simulink model "s_deng_tvg_rev1_13_ramp"  (R2016b)
(part 2 of 19)

      mask prompts: max_pkt_len_bits "Max pkt length, 2^? 64-bit words"; header_ids "SPEAD direct address IDs (decimal)"; header_ind_ids "SPEAD indirect address IDs (decimal)"; spead_msw "SPEAD Flavour (MSw)"; spead_lsw "SPEAD Flavour (LSw)"; spead_version "SPEAD version"; bytes_per_word "Word size, in bytes"
      mask help:
      | This block generates SPEAD-compliant packets from a datastream.
      |
      | Packets are created with a fixed header followed by a number of 64-bit items.
      |
      | Requires a 64-bit data stream.
      |
      | The data_ready signal is one cycle BEFORE valid data! Does not have to be with a valid signal either.
      mask init:
      | if floor(log2(bytes_per_word)) ~= log2(bytes_per_word)
      |     error('Bytes per word should be a power of two.');
      | end
      | 
      | spead_pack_init(gcb)
  spead_pack3 : Subsystem  Tag=casper:spead_pack  AncestorBlock=casper_library_communications/spead_pack  mask(pkt_pack_mask){max_pkt_len_bits=10, header_ids=0x1600, 0x3101, 0x3102, header_ind_ids=0x3300, spead_msw=64, spead_lsw=48, spead_version=4, bytes_per_word=8}
      mask prompts: max_pkt_len_bits "Max pkt length, 2^? 64-bit words"; header_ids "SPEAD direct address IDs (decimal)"; header_ind_ids "SPEAD indirect address IDs (decimal)"; spead_msw "SPEAD Flavour (MSw)"; spead_lsw "SPEAD Flavour (LSw)"; spead_version "SPEAD version"; bytes_per_word "Word size, in bytes"
      mask help:
      | This block generates SPEAD-compliant packets from a datastream.
      |
      | Packets are created with a fixed header followed by a number of 64-bit items.
      |
      | Requires a 64-bit data stream.
      |
      | The data_ready signal is one cycle BEFORE valid data! Does not have to be with a valid signal either.
      mask init:
      | if floor(log2(bytes_per_word)) ~= log2(bytes_per_word)
      |     error('Bytes per word should be a power of two.');
      | end
      | 
      | spead_pack_init(gcb)
  spead_snap0 : Subsystem  Tag=casper:bitsnap  AncestorBlock=casper_library_scopes/bitfield_snapshot  mask(bitsnap){io_names=d64, io_widths=64, io_bps=0, io_types=0, show_format=on, snap_storage=bram, snap_dram_dimm=2, snap_dram_clock=250, snap_nsamples=15, snap_data_width=64, snap_offset=off, snap_circap=off, snap_value=off, snap_ext_arm=off, snap_ext_circ=off, snap_provide_outputs=on, snap_use_dsp48=on, snap_delay=2, extra_names=[c d], extra_widths=[30 2], extra_bps=[0 0], extra_types=[0 0]}
      mask prompts: io_names "Names [msb...lsb]"; io_widths "Bitwidths [msb...lsb]"; io_bps "Binary pts [msb...lsb]"; io_types "Data types [msb...lsb], ufix=0, fix=1, bool=2"; show_format "Print format string?"; snap_storage "Storage medium"; snap_dram_dimm "DRAM dimm"; snap_dram_clock "DRAM clock rate"; snap_nsamples "Number of Samples (2^?)"; snap_data_width "Data width"; snap_offset "Start delay support"; snap_circap "Circular capture support"; snap_value "Extra value capture support"; snap_ext_arm "External arm support"; snap_ext_circ "External circular capture support"; snap_provide_outputs "Provide outputs"; snap_use_dsp48 "Use DSP48s to implement counters"; snap_delay "Pre-snapshot delay"; extra_names "Names [msb...lsb]"; extra_widths "Widths [msb...lsb]"; extra_bps "Binary pts [msb...lsb]"; extra_types "Data types [msb...lsb], ufix=0, fix=1, bool=2"
      mask help:
      | A wrapped snapshot block. Allows specification of inputs to a snapblock word so the toolflow can automatically set up the scope.
      | See documentation for snapshot for explanation of parameters.
      mask init:
      | bitsnap_init(gcb);
      settings: AttributesFormatString=|
      | snap(1):uf64.0 = 64 bits\n64 wide, 32768 deep
      | debugID: 92947725
      mask TypeOptions snap_storage: bram | dram
      mask Callback snap_storage: bitsnap_callback();
      mask TypeOptions snap_dram_dimm: 1 | 2 | 3 | 4
      mask TypeOptions snap_dram_clock: 200 | 250 | 266 | 300 | 333
      mask TypeOptions snap_data_width: 8 | 16 | 32 | 64 | 128
      mask Callback snap_value: bitsnap_callback();
      mask Callback snap_ext_arm: bitsnap_callback();
      mask Callback snap_ext_circ: bitsnap_callback();
      mask Callback snap_provide_outputs: bitsnap_callback();
  speadsnap_control : Subsystem  Tag=xps:sw_reg  AncestorBlock=xps_library/software_register  mask(swreg){io_dir=From Processor, io_delay=0, sample_period=1, names=[speadsnap_arm], bitwidths=1, bin_pts=0, arith_types=2, sim_port=off, show_format=on}
      mask prompts: io_dir "I/O direction"; io_delay "I/O delay"; sample_period "Sample period"; names "Bitfield names [msb...lsb]"; bitwidths "Bitfield widths"; bin_pts "Bitfield binary pts"; arith_types "Bitfield types, ufix=0, fix=1, bool=2"; sim_port "Provide sim input/output?"; show_format "Print format string?"
      mask help: A 32-bit software-accessible register. Can be divided into bitfields of varying widths and types using the fields in the block mask.
      mask init:
      | swreg_init(gcb)
      settings: AttributesFormatString=1input:b = 1 bits
      mask TypeOptions io_dir: To Processor | From Processor
      mask Callback io_dir:
      | mask_enables = get_param(gcb, 'MaskEnables');
      | mask_names = get_param(gcb, 'MaskNames');
      | if strcmp(get_param(gcb, 'io_dir'), 'To Processor'),
      |     mask_enables{ismember(mask_names, 'sample_period')} = 'off';
      | else
      |     mask_enables{ismember(mask_names, 'sample_period')} = 'on';
      | end
      | set_param(gcb, 'MaskEnables', mask_enables);
  speadtime0_offset : Subsystem  Tag=xps:sw_reg  AncestorBlock=xps_library/software register  mask(swreg){io_dir=From Processor, io_delay=1, sample_period=1, names=speadtime_offset0, bitwidths=32, bin_pts=0, arith_types=0, sim_port=on, show_format=on}
      mask prompts: io_dir "I/O direction"; io_delay "I/O delay"; sample_period "Sample period"; names "Bitfield names [msb...lsb]"; bitwidths "Bitfield widths"; bin_pts "Bitfield binary pts"; arith_types "Bitfield types, ufix=0, fix=1, bool=2"; sim_port "Provide sim input/output?"; show_format "Print format string?"
      mask help: A 32-bit software-accessible register. Can be divided into bitfields of varying widths and types using the fields in the block mask.
      mask init:
      | try
      |     swreg_init(gcb)
      | catch ex
      |     disp(sprintf('%s: %s', gcb, ex.message))
      |     errordlg(ex.message)
      | end
      settings: AttributesFormatString=1input:uf32.0 = 32 bits
      mask TypeOptions io_dir: To Processor | From Processor
      mask Callback io_dir:
      | mask_enables = get_param(gcb, 'MaskEnables');
      | mask_names = get_param(gcb, 'MaskNames');
      | if strcmp(get_param(gcb, 'io_dir'), 'To Processor'),
      |     mask_enables{ismember(mask_names, 'sample_period')} = 'off';
      | else
      |     mask_enables{ismember(mask_names, 'sample_period')} = 'on';
      | end
      | set_param(gcb, 'MaskEnables', mask_enables);
  speadtime1_offset : Subsystem  Tag=xps:sw_reg  AncestorBlock=xps_library/software register  mask(swreg){io_dir=From Processor, io_delay=1, sample_period=1, names=speadtime_offset1, bitwidths=32, bin_pts=0, arith_types=0, sim_port=on, show_format=on}
      mask prompts: io_dir "I/O direction"; io_delay "I/O delay"; sample_period "Sample period"; names "Bitfield names [msb...lsb]"; bitwidths "Bitfield widths"; bin_pts "Bitfield binary pts"; arith_types "Bitfield types, ufix=0, fix=1, bool=2"; sim_port "Provide sim input/output?"; show_format "Print format string?"
      mask help: A 32-bit software-accessible register. Can be divided into bitfields of varying widths and types using the fields in the block mask.
      mask init:
      | try
      |     swreg_init(gcb)
      | catch ex
      |     disp(sprintf('%s: %s', gcb, ex.message))
      |     errordlg(ex.message)
      | end
      settings: AttributesFormatString=1input:uf32.0 = 32 bits
      mask TypeOptions io_dir: To Processor | From Processor
      mask Callback io_dir:
      | mask_enables = get_param(gcb, 'MaskEnables');
      | mask_names = get_param(gcb, 'MaskNames');
      | if strcmp(get_param(gcb, 'io_dir'), 'To Processor'),
      |     mask_enables{ismember(mask_names, 'sample_period')} = 'off';
      | else
      |     mask_enables{ismember(mask_names, 'sample_period')} = 'on';
      | end
      | set_param(gcb, 'MaskEnables', mask_enables);
  start_flag_lsw : Subsystem  Tag=xps:sw_reg  AncestorBlock=xps_library/software register  mask(swreg){io_dir=From Processor, io_delay=1, sample_period=1, names=reg, bitwidths=32, bin_pts=0, arith_types=0, sim_port=on, show_format=on}
      mask prompts: io_dir "I/O direction"; io_delay "I/O delay"; sample_period "Sample period"; names "Bitfield names [msb...lsb]"; bitwidths "Bitfield widths"; bin_pts "Bitfield binary pts"; arith_types "Bitfield types, ufix=0, fix=1, bool=2"; sim_port "Provide sim input/output?"; show_format "Print format string?"
      mask help: A 32-bit software-accessible register. Can be divided into bitfields of varying widths and types using the fields in the block mask.
      mask init:
      | try
      |     swreg_init(gcb)
      | catch ex
      |     disp(sprintf('%s: %s', gcb, ex.message))
      |     errordlg(ex.message)
      | end
      settings: AttributesFormatString=1input:uf32.0 = 32 bits
      mask TypeOptions io_dir: To Processor | From Processor
      mask Callback io_dir:
      | mask_enables = get_param(gcb, 'MaskEnables');
      | mask_names = get_param(gcb, 'MaskNames');
      | if strcmp(get_param(gcb, 'io_dir'), 'To Processor'),
      |     mask_enables{ismember(mask_names, 'sample_period')} = 'off';
      | else
      |     mask_enables{ismember(mask_names, 'sample_period')} = 'on';
      | end
      | set_param(gcb, 'MaskEnables', mask_enables);
  start_flag_msw : Subsystem  Tag=xps:sw_reg  AncestorBlock=xps_library/software register  mask(swreg){io_dir=From Processor, io_delay=1, sample_period=1, names=reg, bitwidths=32, bin_pts=0, arith_types=0, sim_port=on, show_format=on}
      mask prompts: io_dir "I/O direction"; io_delay "I/O delay"; sample_period "Sample period"; names "Bitfield names [msb...lsb]"; bitwidths "Bitfield widths"; bin_pts "Bitfield binary pts"; arith_types "Bitfield types, ufix=0, fix=1, bool=2"; sim_port "Provide sim input/output?"; show_format "Print format string?"
      mask help: A 32-bit software-accessible register. Can be divided into bitfields of varying widths and types using the fields in the block mask.
      mask init:
      | try
      |     swreg_init(gcb)
      | catch ex
      |     disp(sprintf('%s: %s', gcb, ex.message))
      |     errordlg(ex.message)
      | end
      settings: AttributesFormatString=1input:uf32.0 = 32 bits
      mask TypeOptions io_dir: To Processor | From Processor
      mask Callback io_dir:
      | mask_enables = get_param(gcb, 'MaskEnables');
      | mask_names = get_param(gcb, 'MaskNames');
      | if strcmp(get_param(gcb, 'io_dir'), 'To Processor'),
      |     mask_enables{ismember(mask_names, 'sample_period')} = 'off';
      | else
      |     mask_enables{ismember(mask_names, 'sample_period')} = 'on';
      | end
      | set_param(gcb, 'MaskEnables', mask_enables);
  start_time_lsw : Subsystem  Tag=xps:sw_reg  AncestorBlock=xps_library/software register  mask(swreg){io_dir=From Processor, io_delay=1, sample_period=1, names=reg, bitwidths=32, bin_pts=0, arith_types=0, sim_port=on, show_format=on}
      mask prompts: io_dir "I/O direction"; io_delay "I/O delay"; sample_period "Sample period"; names "Bitfield names [msb...lsb]"; bitwidths "Bitfield widths"; bin_pts "Bitfield binary pts"; arith_types "Bitfield types, ufix=0, fix=1, bool=2"; sim_port "Provide sim input/output?"; show_format "Print format string?"
      mask help: A 32-bit software-accessible register. Can be divided into bitfields of varying widths and types using the fields in the block mask.
      mask init:
      | try
      |     swreg_init(gcb)
      | catch ex
      |     disp(sprintf('%s: %s', gcb, ex.message))
      |     errordlg(ex.message)
      | end
      settings: AttributesFormatString=1input:uf32.0 = 32 bits
      mask TypeOptions io_dir: To Processor | From Processor
      mask Callback io_dir:
      | mask_enables = get_param(gcb, 'MaskEnables');
      | mask_names = get_param(gcb, 'MaskNames');
      | if strcmp(get_param(gcb, 'io_dir'), 'To Processor'),
      |     mask_enables{ismember(mask_names, 'sample_period')} = 'off';
      | else
      |     mask_enables{ismember(mask_names, 'sample_period')} = 'on';
      | end
      | set_param(gcb, 'MaskEnables', mask_enables);
  start_time_msw : Subsystem  Tag=xps:sw_reg  AncestorBlock=xps_library/software register  mask(swreg){io_dir=From Processor, io_delay=1, sample_period=1, names=reg, bitwidths=32, bin_pts=0, arith_types=0, sim_port=on, show_format=on}
      mask prompts: io_dir "I/O direction"; io_delay "I/O delay"; sample_period "Sample period"; names "Bitfield names [msb...lsb]"; bitwidths "Bitfield widths"; bin_pts "Bitfield binary pts"; arith_types "Bitfield types, ufix=0, fix=1, bool=2"; sim_port "Provide sim input/output?"; show_format "Print format string?"
      mask help: A 32-bit software-accessible register. Can be divided into bitfields of varying widths and types using the fields in the block mask.
      mask init:
      | try
      |     swreg_init(gcb)
      | catch ex
      |     disp(sprintf('%s: %s', gcb, ex.message))
      |     errordlg(ex.message)
      | end
      settings: AttributesFormatString=1input:uf32.0 = 32 bits
      mask TypeOptions io_dir: To Processor | From Processor
      mask Callback io_dir:
      | mask_enables = get_param(gcb, 'MaskEnables');
      | mask_names = get_param(gcb, 'MaskNames');
      | if strcmp(get_param(gcb, 'io_dir'), 'To Processor'),
      |     mask_enables{ismember(mask_names, 'sample_period')} = 'off';
      | else
      |     mask_enables{ismember(mask_names, 'sample_period')} = 'on';
      | end
      | set_param(gcb, 'MaskEnables', mask_enables);
  test_control : Subsystem  Tag=xps:sw_reg  AncestorBlock=xps_library/software_register  mask(swreg){io_dir=From Processor, io_delay=0, sample_period=1, names=[sel_ramp80 rst_ramp80 sel_munge], bitwidths=1, bin_pts=0, arith_types=2, sim_port=off, show_format=on}
      mask prompts: io_dir "I/O direction"; io_delay "I/O delay"; sample_period "Sample period"; names "Bitfield names [msb...lsb]"; bitwidths "Bitfield widths"; bin_pts "Bitfield binary pts"; arith_types "Bitfield types, ufix=0, fix=1, bool=2"; sim_port "Provide sim input/output?"; show_format "Print format string?"
      mask help: A 32-bit software-accessible register. Can be divided into bitfields of varying widths and types using the fields in the block mask.
      mask init:
      | swreg_init(gcb)
      settings: AttributesFormatString=3 inputs:b,b,b = 3 bits
      mask TypeOptions io_dir: To Processor | From Processor
      mask Callback io_dir:
      | mask_enables = get_param(gcb, 'MaskEnables');
      | mask_names = get_param(gcb, 'MaskNames');
      | if strcmp(get_param(gcb, 'io_dir'), 'To Processor'),
      |     mask_enables{ismember(mask_names, 'sample_period')} = 'off';
      | else
      |     mask_enables{ismember(mask_names, 'sample_period')} = 'on';
      | end
      | set_param(gcb, 'MaskEnables', mask_enables);
  tick_offset_lsw : Subsystem  Tag=xps:sw_reg  AncestorBlock=xps_library/software register  mask(swreg){io_dir=From Processor, io_delay=1, sample_period=1, names=reg, bitwidths=32, bin_pts=0, arith_types=0, sim_port=off, show_format=on}
      mask prompts: io_dir "I/O direction"; io_delay "I/O delay"; sample_period "Sample period"; names "Bitfield names [msb...lsb]"; bitwidths "Bitfield widths"; bin_pts "Bitfield binary pts"; arith_types "Bitfield types, ufix=0, fix=1, bool=2"; sim_port "Provide sim input/output?"; show_format "Print format string?"
      mask help: A 32-bit software-accessible register. Can be divided into bitfields of varying widths and types using the fields in the block mask.
      mask init:
      | try
      |     swreg_init(gcb)
      | catch ex
      |     disp(sprintf('%s: %s', gcb, ex.message))
      |     errordlg(ex.message)
      | end
      settings: AttributesFormatString=1input:uf32.0 = 32 bits
      mask TypeOptions io_dir: To Processor | From Processor
      mask Callback io_dir:
      | mask_enables = get_param(gcb, 'MaskEnables');
      | mask_names = get_param(gcb, 'MaskNames');
      | if strcmp(get_param(gcb, 'io_dir'), 'To Processor'),
      |     mask_enables{ismember(mask_names, 'sample_period')} = 'off';
      | else
      |     mask_enables{ismember(mask_names, 'sample_period')} = 'on';
      | end
      | set_param(gcb, 'MaskEnables', mask_enables);
  tick_offset_msw : Subsystem  Tag=xps:sw_reg  AncestorBlock=xps_library/software register  mask(swreg){io_dir=From Processor, io_delay=1, sample_period=1, names=reg, bitwidths=32, bin_pts=0, arith_types=0, sim_port=off, show_format=on}
      mask prompts: io_dir "I/O direction"; io_delay "I/O delay"; sample_period "Sample period"; names "Bitfield names [msb...lsb]"; bitwidths "Bitfield widths"; bin_pts "Bitfield binary pts"; arith_types "Bitfield types, ufix=0, fix=1, bool=2"; sim_port "Provide sim input/output?"; show_format "Print format string?"
      mask help: A 32-bit software-accessible register. Can be divided into bitfields of varying widths and types using the fields in the block mask.
      mask init:
      | try
      |     swreg_init(gcb)
      | catch ex
      |     disp(sprintf('%s: %s', gcb, ex.message))
      |     errordlg(ex.message)
      | end
      settings: AttributesFormatString=1input:uf32.0 = 32 bits
      mask TypeOptions io_dir: To Processor | From Processor
      mask Callback io_dir:
      | mask_enables = get_param(gcb, 'MaskEnables');
      | mask_names = get_param(gcb, 'MaskNames');
      | if strcmp(get_param(gcb, 'io_dir'), 'To Processor'),
      |     mask_enables{ismember(mask_names, 'sample_period')} = 'off';
      | else
      |     mask_enables{ismember(mask_names, 'sample_period')} = 'on';
      | end
      | set_param(gcb, 'MaskEnables', mask_enables);
  ticks_since_mrst : Subsystem
  tvg_spead_time_with_pkt_ctr : Subsystem  mask{packetlen_bits=9}
      mask prompts: packetlen_bits "Packet length, num 80-bit words (2^?):"
  wr_addr{0..3} (4 alike) : xbsIndex_r4/Counter  cnt_type=Free Running  cnt_to=Inf  operation=Up  start_count=0  cnt_by_val=1  arith_type=Unsigned  n_bits=10  bin_pt=0  load_pin=off  rst=on  en=on  explicit_period=on  period=1  use_behavioral_HDL=off  implementation=Fabric  dbl_ovrd=off  block_type=counter
  tag scope: local_time=global
  wires:
  bus_create4/1(bus_out) -> Assert/1  "d80_0"
  fifo0/1(fifo_data80) -> pipeline96/1(d)  "data00"
  fifo0/2(fifo_dv) -> pipeline97/1(d)  "dv00"
  fifo0/3(word_start) -> pipeline98/1(d)  "ws00"
  fifo0/4(pkt_start) -> pipeline99/1(d)  "ps00"
  gbe_porttx/1(in_reg) -> pipeline15/1(d)
  Constant9/1 -> gbe_porttx/1(sim_1)
  Constant10/1 -> gbe_iptx0/1(sim_1)
  Constant12/1 -> gbe_iptx1/1(sim_1)
  Constant13/1 -> gbe_iptx2/1(sim_1)
  Constant14/1 -> gbe_iptx3/1(sim_1)
  Constant15/1 -> digitiser_id/1(sim_1)
  Constant17/1 -> receptor_id/1(sim_1)
  fifo0/5(fifo_full) -> Terminator16/1  "full00"
  fifo0/6(fifo_empty) -> Terminator23/1  "empty00"
  fifo1/1(fifo_data80) -> pipeline100/1(d)  "data01"
  fifo1/2(fifo_dv) -> pipeline101/1(d)  "dv01"
  fifo1/3(word_start) -> pipeline102/1(d)  "ws01"
  fifo1/4(pkt_start) -> pipeline103/1(d)  "ps01"
  pack_80_64_1/2(valid64) -> pipeline116/1(d)  "v64_01"
  pack_80_64_1/1(ready64) -> pipeline115/1(d)  "r64_01"
  fifo1/5(fifo_full) -> Terminator18/1
  fifo1/6(fifo_empty) -> Terminator20/1
  Constant16/1 -> digitiser_id/2(sim_2)
  receptor_id/1(in_receptor_id) -> bus_create/3(in3)
  Constant6/1 -> receptor_id/2(sim_2)
  Constant19/1 -> receptor_id/3(sim_3)
  [hdr_0x3101] -> bus_create9/1(in1)
  [pol0_id] -> bus_create9/2(in2)
  [hdr_0x3101] -> bus_create1/1(in1)
  [pol0_id] -> bus_create1/2(in2)
  [speadtime0] -> spead_pack0/8(hdr5_0x1600_DIR), spead_pack0/4(hdr_heap_id)  "timein0"
  bus_create9/1(bus_out) -> spead_pack0/9(hdr6_0x3101_DIR)
  [status0] -> spead_pack0/10(hdr7_0x3102_DIR)
  bus_create1/1(bus_out) -> spead_pack1/9(hdr6_0x3101_DIR)
  [status1] -> spead_pack1/10(hdr7_0x3102_DIR)
  [tvg_ltime] -> fifo_select/1(localtime)
  fifo_select/1(select) -> Delay3/1  "fifo_select"
  Delay3/1 -> fifo0/2(fifo_we_en), [fifoselect], Inverter/1  "fifoselect"
  [speadtime1] -> spead_pack1/4(hdr_heap_id), spead_pack1/8(hdr5_0x1600_DIR)  "timein1"
  pack_80_64_00/1(ready64) -> pipeline112/1(d)  "r64_00"
  pack_80_64_00/2(valid64) -> pipeline113/1(d)  "v64_00"
  [spead_heapsize] -> spead_pack0/5(hdr_heap_size)
  [spead_heapoffset] -> spead_pack0/6(hdr_heap_offset)
  [spead_pktlen] -> spead_pack0/7(hdr_pkt_len_words)
  [spead_heapsize] -> spead_pack1/5(hdr_heap_size)
  [spead_heapoffset] -> spead_pack1/6(hdr_heap_offset)
  [spead_pktlen] -> spead_pack1/7(hdr_pkt_len_words)
  [masked_time] -> Delay128/1
  Assert/1 -> fifo1/1(data80), fifo0/1(data80)
  tvg_spead_time_with_pkt_ctr/1(local_time) -> Delay131/1
  tvg_spead_time_with_pkt_ctr/2(spead_time) -> Delay132/1
  spead_pack1/4(data_overflow) -> Terminator15/1
  [adc_data_offset] -> spead_pack0/11(hdr8_0x3300)
  [adc_data_offset] -> spead_pack1/11(hdr8_0x3300)
  Constant26/1 -> [spead_heapsize]
  Constant27/1 -> [spead_pktlen]
  Constant45/1 -> [spead_heapoffset]
  spead_pack0/4(data_overflow) -> Terminator12/1
  spead_pack0/3(eof) -> pipeline56/1(d)
  spead_pack0/1(data_out) -> pipeline54/1(d)  "packd"
  spead_pack0/2(valid_out) -> pipeline55/1(d)  "packv"
  spead_pack1/1(data_out) -> pipeline57/1(d)
  spead_pack1/2(valid_out) -> pipeline58/1(d)
  spead_pack1/3(eof) -> pipeline59/1(d)
  [fifoselect] -> edge_detect5/1(in), Inverter2/1
  Register5/1 -> [speadtime0]  "speadtime0"
  Inverter2/1 -> edge_detect6/1(in)
  edge_detect5/1(out) -> Register5/2
  edge_detect6/1(out) -> Register6/2
  Register6/1 -> [speadtime1]  "speadtime1"
  Constant8/1 -> [adc_data_offset]
  [mrst] -> ticks_since_mrst/1(reset)
  [sync] -> ticks_since_mrst/2(sync)
  ticks_since_mrst/1(time64) -> [local_time]  "localtime"
  [msync] -> [sync]  "sync"
  edge_detect2/1(out) -> [mrst]  "mrst"
  edge_detect1/1(out) -> [msync]  "msync"
  edge_detect4/1(out) -> [clr_status]  "clr_status"
  [local_time] -> slice1/1, slice2/1
  Constant28/1 -> control/3(sim_3)
  Constant44/1 -> control/1(sim_1)
  Constant24/1 -> control/2(sim_2)
  Constant33/1 -> control/6(sim_6)
  Constant30/1 -> control/5(sim_5)
  Constant36/1 -> control/4(sim_4)
  Pulse Generator/1 -> control/8(sim_8)
  [tick_offset] -> ticks_since_mrst/3(offset)
  edge_detect10/1(out) -> [load_tick_offset]  "mrst"
  Constant20/1 -> control/9(sim_9)
  digitiser_id/1(in_digitiser_serial) -> bus_create/1(in1)
  digitiser_id/2(in_digitiser_type) -> bus_create/2(in2)
  Constant43/1 -> flag_setup/3(sim_3)
  Constant42/1 -> flag_setup/2(sim_2)
  Constant39/1 -> flag_setup/1(sim_1)
  Counter Free-Running3/1 -> Relational Operator4/2
  Constant48/1 -> Relational Operator4/1
  Relational Operator4/1 -> flag_setup/4(sim_4)
  Constant52/1 -> start_flag_msw/1(sim_1)
  Constant53/1 -> start_flag_lsw/1(sim_1)
  Constant51/1 -> end_flag_msw/1(sim_1)
  Constant50/1 -> end_flag_lsw/1(sim_1)
  Concat4/1 -> Delay49/1  "starttime"
  Concat5/1 -> Delay50/1  "stoptime"
  [flag_start_time] -> Delay46/1
  [local_time] -> Delay45/1, Delay47/1
  [flag_end_time] -> Delay48/1, Delay51/1
  Relational/1 -> Logical2/2  "start_okay"
  [flag_armed] -> Delay44/1
  Relational1/1 -> Logical4/2  "end_okay"
  Logical2/1 -> Delay23/1  "start_okay"
  Logical4/1 -> Logical3/1  "end_okay"
  edge_detect9/1(out) -> [load_flag_time]  "loadtimes"
  Constant4/1 -> Register1/1
  edge_detect8/1(out) -> [reset_flag_time]  "rst"
  [reset_flag_time] -> Register1/2
  [load_flag_time] -> Register1/3
  Register1/1 -> [flag_armed]  "armed"
  Relational Operator3/1 -> flag_setup/5(sim_5)
  Relational2/1 -> Delay22/1  "zero_stop"
  Constant2/1 -> Relational2/2
  Logical3/1 -> Logical1/2  "eokay"
  Counter Free-Running2/1 -> Relational Operator3/2
  Constant5/1 -> Relational Operator3/1
  Logical5/1 -> sample_masking/2(den_in)
  Constant49/1 -> start_time_msw/1(sim_1)
  Constant54/1 -> start_time_lsw/1(sim_1)
  Constant3/1 -> end_time_msw/1(sim_1)
  Constant11/1 -> end_time_lsw/1(sim_1)
  Relational3/1 -> Logical6/2  "start_okay"
  Relational4/1 -> Logical8/2  "end_okay"
  [start_time] -> Delay39/1
  Relational6/1 -> Delay15/1  "first_sample"
  [end_time] -> Delay41/1
  Relational7/1 -> Delay16/1  "last_sample"
  [sample_end] -> sample_masking/6(sample_end)
  [sample_start] -> sample_masking/5(sample_start)
  sample_masking/2(den_out) -> Delay126/1  "enable"
  sample_masking/3(data_mask) -> Delay127/1  "mask"
  edge_detect11/1(out) -> [reset_en_time]  "reset_en_time"
  Relational Operator5/1 -> control_output/2(sim_2)
  Counter Free-Running4/1 -> Relational Operator6/2, Relational Operator5/2
  Constant38/1 -> Relational Operator5/1
  edge_detect12/1(out) -> [load_en_time]  "load_en_time"
  Concat/1 -> Delay42/1
  Concat1/1 -> Delay43/1
  Constant22/1 -> Register2/1
  [reset_en_time] -> Register2/2
  [load_en_time] -> Register2/3
  Register2/1 -> [en_armed]  "armed"
  Logical6/1 -> Delay17/1  "start_okay"
  Logical8/1 -> Logical7/1  "end_okay"
  Logical7/1 -> Logical5/2
  Constant34/1 -> Delay37/1
  Relational5/1 -> Delay14/1
  Constant29/1 -> control_output/3(sim_3)
  Constant47/1 -> control_output/4(sim_4)
  Constant31/1 -> Relational Operator6/1
  Relational Operator6/1 -> control_output/1(sim_1)
  [data_enable] -> Delay129/1
  [sample_mask] -> Delay130/1
  Concat2/1 -> Register3/1
  [load_tick_offset] -> Register3/2
  Register3/1 -> [tick_offset]
  pipeline21/1(q) -> edge_detect12/1(in)
  pipeline22/1(q) -> edge_detect11/1(in)
  pipeline23/1(q) -> [sample_start]
  pipeline24/1(q) -> [sample_end]
  Delay42/1 -> [start_time]
  Delay43/1 -> [end_time]
  Delay49/1 -> [flag_start_time]
  Delay50/1 -> [flag_end_time]
  pipeline10/1(q) -> [gbe_ip3]
  pipeline11/1(q) -> [gbe_ip2]
  pipeline13/1(q) -> [gbe_ip0]
  pipeline9/1(q) -> [gbe_port]
  Delay126/1 -> [data_enable]
  Delay127/1 -> [sample_mask]
  Delay128/1 -> tvg_spead_time_with_pkt_ctr/1(localtime64)
  Delay129/1 -> tvg_spead_time_with_pkt_ctr/2(data_enable)
  Delay130/1 -> tvg_spead_time_with_pkt_ctr/3(data_mask)
  Delay131/1 -> [tvg_ltime]
  Delay132/1 -> [tvg_stime]
  pipeline25/1(q) -> Concat/1
  pipeline26/1(q) -> Concat/2
  pipeline27/1(q) -> Concat1/1
  pipeline28/1(q) -> Concat1/2
  pipeline29/1(q) -> [hdr_0x3101]
  pipeline30/1(q) -> [pol0_id]
  pipeline31/1(q) -> [pol1_id]
  control/1(in_up_cnt_rst) -> pipeline/1(d)
  pipeline/1(q) -> edge_detect3/1(in)
  control/2(in_tvg_select0) -> pipeline1/1(d)
  control/3(in_tvg_select1) -> pipeline2/1(d)
  control/4(in_clr_status) -> pipeline3/1(d)
  control/5(in_gbe_rst) -> pipeline4/1(d)
  control/6(in_gbe_txen) -> pipeline5/1(d)
  control/7(in_msync) -> pipeline6/1(d)
  control/8(in_mrst) -> pipeline7/1(d)
  control/9(in_load_tick_offset) -> pipeline8/1(d)
  pipeline8/1(q) -> edge_detect10/1(in)
  pipeline7/1(q) -> edge_detect2/1(in)
  pipeline6/1(q) -> edge_detect1/1(in)
  pipeline4/1(q) -> [gbe_rst]
  pipeline3/1(q) -> edge_detect4/1(in)
  pipeline12/1(q) -> [gbe_ip1]
  gbe_iptx0/1(in_reg) -> pipeline13/1(d)
  gbe_iptx1/1(in_reg) -> pipeline12/1(d)
  gbe_iptx2/1(in_reg) -> pipeline11/1(d)
  gbe_iptx3/1(in_reg) -> pipeline10/1(d)
  pipeline17/1(q) -> Concat2/1
  tick_offset_lsw/1(in_reg) -> pipeline18/1(d)
  pipeline18/1(q) -> Concat2/2
  slice1/1 -> pipeline20/1(d)
  pipeline20/1(q) -> local_time_lsw/1(out_reg)
  slice2/1 -> pipeline19/1(d)
  pipeline19/1(q) -> local_time_msw/1(out_reg)
  end_time_lsw/1(in_reg) -> pipeline28/1(d)
  end_time_msw/1(in_reg) -> pipeline27/1(d)
  start_time_lsw/1(in_reg) -> pipeline26/1(d)
  start_time_msw/1(in_reg) -> pipeline25/1(d)
  control_output/4(in_sample_end) -> pipeline24/1(d)
  control_output/3(in_sample_start) -> pipeline23/1(d)
  control_output/2(in_reset_en_time) -> pipeline22/1(d)
  control_output/1(in_load_en_time) -> pipeline21/1(d)
  bus_create/1(bus_out) -> pipeline29/1(d)
  receptor_id/2(in_pol0_id) -> pipeline30/1(d)
  receptor_id/3(in_pol1_id) -> pipeline31/1(d)
  flag_setup/1(in_adc_count) -> pipeline32/1(d)
  flag_setup/2(in_adc_flag) -> pipeline33/1(d)
  flag_setup/3(in_ndiode_flag) -> pipeline34/1(d)
  flag_setup/4(in_load_flags) -> pipeline35/1(d)
  flag_setup/5(in_reset_flags) -> pipeline36/1(d)
  pipeline36/1(q) -> edge_detect8/1(in)
  pipeline35/1(q) -> edge_detect9/1(in)
  pipeline34/1(q) -> [ndiode_flag]
  pipeline33/1(q) -> [adc_flag]
  pipeline32/1(q) -> [adc_count]
  start_flag_msw/1(in_reg) -> pipeline37/1(d)
  pipeline37/1(q) -> Concat4/1
  start_flag_lsw/1(in_reg) -> pipeline38/1(d)
  pipeline38/1(q) -> Concat4/2
  end_flag_msw/1(in_reg) -> pipeline39/1(d)
  pipeline39/1(q) -> Concat5/1
  end_flag_lsw/1(in_reg) -> pipeline40/1(d)
  pipeline40/1(q) -> Concat5/2
  pipeline54/1(q) -> [spead_data0]
  pipeline55/1(q) -> [spead_valid0]  "sp_dv0"
  pipeline56/1(q) -> [spead_eof0]
  pipeline57/1(q) -> [spead_data1]
  pipeline58/1(q) -> [spead_valid1]  "sp_dv1"
  pipeline59/1(q) -> [spead_eof1]
  pipeline96/1(q) -> Mux12/2  "d80"
  pipeline97/1(q) -> pack_80_64_00/2(valid80)  "v80"
  pipeline98/1(q) -> pack_80_64_00/3(word_start)  "wd_start"
  pipeline99/1(q) -> Delay7/1, pack_80_64_00/4(pkt_start)  "pkt_start"
  pipeline100/1(q) -> Mux13/2
  pipeline101/1(q) -> pack_80_64_1/2(valid80)
  pipeline102/1(q) -> pack_80_64_1/3(word_start)
  pipeline103/1(q) -> Delay8/1, pack_80_64_1/4(pkt_start)
  pipeline112/1(q) -> [rdy0], spead_pack0/1(data64_ready)
  pipeline113/1(q) -> [vld0], spead_pack0/2(data64_valid)
  pipeline115/1(q) -> [rdy1], spead_pack1/1(data64_ready)
  pipeline116/1(q) -> [vld1], spead_pack1/2(data64_valid)
  pipeline15/1(q) -> pipeline9/1(d)
  Delay13/1 -> Logical8/1, Logical6/1
  Delay14/1 -> Logical7/2
  Delay15/1 -> Delay18/1
  Delay16/1 -> Delay19/1
  Delay17/1 -> Logical5/1
  Delay18/1 -> Delay20/1
  Delay19/1 -> Delay21/1
  Delay20/1 -> sample_masking/3(first_samples)
  Delay21/1 -> sample_masking/4(last_samples)
  Delay22/1 -> Logical3/2
  Delay23/1 -> Logical1/1
  Delay24/1 -> Delay25/1
  Delay25/1 -> Delay26/1
  Delay26/1 -> Delay27/1
  Delay27/1 -> sample_masking/1(timei)
  sample_masking/4(flag_valid) -> Delay28/1
  Delay28/1 -> [flag_en]
  Logical1/1 -> sample_masking/7(flag_en)  "flag_en"
  sample_masking/1(timeo) -> Delay29/1
  Delay29/1 -> [masked_time]
  [local_time] -> Delay30/1
  [en_armed] -> Delay31/1
  [local_time] -> Delay32/1, Delay34/1, Delay38/1, Delay40/1
  [start_time] -> Delay33/1
  [end_time] -> Delay35/1, Delay36/1
  Delay30/1 -> Delay24/1
  Delay31/1 -> Delay13/1
  Delay32/1 -> Relational3/1
  Delay33/1 -> Relational3/2
  Delay34/1 -> Relational4/1
  Delay35/1 -> Relational4/2
  Delay36/1 -> Relational5/1
  Delay37/1 -> Relational5/2
  Delay38/1 -> Relational6/1
  Delay39/1 -> Relational6/2
  Delay40/1 -> Relational7/1
  Delay41/1 -> Relational7/2
  Delay44/1 -> Logical4/1, Logical2/1
  Delay45/1 -> Relational/1
  Delay46/1 -> Relational/2
  Delay47/1 -> Relational1/1
  Delay48/1 -> Relational1/2
  Delay51/1 -> Relational2/1
  Pulse Generator1/1 -> control/7(sim_7)
  pipeline5/1(q) -> Terminator49/1
  edge_detect3/1(out) -> Terminator50/1  "mrst"
  AddSub/1 -> Slice/1
  AddSub1/1 -> Slice1/1
  [tvg_stime] -> AddSub1/1, AddSub/1
  Constant81/1 -> speadtime0_offset/1(sim_1)
  Slice/1 -> Register5/1
  Slice1/1 -> Register6/1
  speadtime0_offset/1(in_speadtime_offset0) -> AddSub/2
  Constant82/1 -> speadtime1_offset/1(sim_1)
  speadtime1_offset/1(in_speadtime_offset1) -> AddSub1/2
  Inverter/1 -> fifo1/2(fifo_we_en)
  [adc_count] -> Concat6/1
  Constant90/1 -> Concat6/2
  Delay4/1 -> [status0]
  Delay55/1 -> [status3]
  Delay54/1 -> [status2]
  Delay53/1 -> [status1]
  Concat6/1 -> Delay4/1, Delay53/1, Delay54/1, Delay55/1
  [ndiode_flag] -> Convert28/1
  Logical/1 -> Convert27/1
  Logical19/1 -> Convert30/1
  [adc_flag] -> Convert29/1
  [flag_en] -> Logical/1, Logical19/2
  Convert28/1 -> Logical/2
  Convert29/1 -> Logical19/1
  Convert30/1 -> Concat6/3
  Convert27/1 -> Concat6/4
  tick_offset_msw/1(in_reg) -> pipeline17/1(d)
  gbecontrol/1(in_gbe0) -> [gbe_txen0]
  gbecontrol/2(in_gbe1) -> [gbe_txen1]
  gbecontrol/3(in_gbe2) -> [gbe_txen2]
  gbecontrol/4(in_gbe3) -> [gbe_txen3]
  ramp0/1 -> [rampdata0]
  [vld0] -> ramp0/2
  [rdy0] -> ramp0/1
  ramp1/1 -> [rampdata1]
  [vld1] -> ramp1/2
  [rdy1] -> ramp1/1
  [spead_data0] -> spead_snap0/1(in_d64)
  [spead_valid0] -> spead_snap0/2(we)
  [spead_eof0] -> spead_detail/1(in_eof)
  [spead_valid0] -> spead_detail/2(in_we), spead_detail/3(we)
  Logical37/1 -> spead_detail/4(trig), spead_snap0/3(trig)
  [spead_eof0] -> Logical37/2
  [speadsnap_arm] -> Logical37/1
  speadsnap_control/1(in_speadsnap_arm) -> Delay1/1
  Delay1/1 -> [speadsnap_arm]
  Mux8/1 -> spead_pack0/3(data64)
  Mux9/1 -> spead_pack1/3(data64)
  [spead_data0] -> pipeline16/1(d)
  [spead_valid0] -> pipeline41/1(d)
  wr_addr0/1 -> 64_to_256/1  "waddr"
  [spead_valid0] -> edge_detect7/1(in), edge_detect/1, pipeline14/1(d)
  Constant57/1 -> 64_to_256/6
  Constant58/1 -> 64_to_256/5
  rd_addr0/1 -> 64_to_256/4, Relational8/2  "rdaddr"
  edge_detect/1 -> wr_addr0/1
  pipeline14/1(q) -> wr_addr0/2
  pipeline16/1(q) -> 64_to_256/2
  pipeline41/1(q) -> 64_to_256/3  "dv64_0"
  64_to_256/1 -> Terminator7/1
  edge_detect7/1(out) -> rd_addr0/1, rd_arm/3, rd_arm/1
  Constant7/1 -> Relational8/1
  Relational8/1 -> rd_arm/2  "rd_done"
  rd_arm/1 -> pipeline42/1(d), rd_addr0/2  "rd_en"
  pipeline42/1(q) -> pipeline43/1(d), edge_detect13/1(in)
  edge_detect13/1(out) -> [sp256_eof0]  "eof256_0"
  bus_create5/1(bus_out) -> Assert1/1  "d80_0"
  fifo2/1(fifo_data80) -> pipeline65/1(d)  "data00"
  fifo2/2(fifo_dv) -> pipeline66/1(d)  "dv00"
  fifo2/3(word_start) -> pipeline67/1(d)  "ws00"
  fifo2/4(pkt_start) -> pipeline68/1(d)  "ps00"
  fifo2/5(fifo_full) -> Terminator3/1  "full00"
  fifo2/6(fifo_empty) -> Terminator6/1  "empty00"
  fifo3/1(fifo_data80) -> pipeline45/1(d)  "data01"
  fifo3/2(fifo_dv) -> pipeline46/1(d)  "dv01"
  fifo3/3(word_start) -> pipeline47/1(d)  "ws01"
  fifo3/4(pkt_start) -> pipeline48/1(d)  "ps01"
  pack_80_64_3/2(valid64) -> pipeline52/1(d)  "v64_01"
  pack_80_64_3/1(ready64) -> pipeline51/1(d)  "r64_01"
  fifo3/5(fifo_full) -> Terminator4/1
  fifo3/6(fifo_empty) -> Terminator5/1
  [hdr_0x3101] -> bus_create3/1(in1)
  [pol1_id] -> bus_create3/2(in2)
  [hdr_0x3101] -> bus_create2/1(in1)
  [pol1_id] -> bus_create2/2(in2)
  [speadtime0] -> spead_pack2/4(hdr_heap_id), spead_pack2/8(hdr5_0x1600_DIR)  "timein0"
  bus_create3/1(bus_out) -> spead_pack2/9(hdr6_0x3101_DIR)
  [status2] -> spead_pack2/10(hdr7_0x3102_DIR)
  bus_create2/1(bus_out) -> spead_pack3/9(hdr6_0x3101_DIR)
  [status3] -> spead_pack3/10(hdr7_0x3102_DIR)
  [tvg_ltime] -> fifo_select1/1(localtime)
  fifo_select1/1(select) -> Delay2/1  "fifo_select"
  Delay2/1 -> Inverter1/1, fifo2/2(fifo_we_en)  "fifoselect"
  [speadtime1] -> spead_pack3/8(hdr5_0x1600_DIR), spead_pack3/4(hdr_heap_id)  "timein1"
  pack_80_64_2/1(ready64) -> pipeline49/1(d)  "r64_00"
  pack_80_64_2/2(valid64) -> pipeline50/1(d)  "v64_00"
  [spead_heapsize] -> spead_pack2/5(hdr_heap_size)
  [spead_heapoffset] -> spead_pack2/6(hdr_heap_offset)
  [spead_pktlen] -> spead_pack2/7(hdr_pkt_len_words)
  [spead_heapsize] -> spead_pack3/5(hdr_heap_size)
  [spead_heapoffset] -> spead_pack3/6(hdr_heap_offset)
  [spead_pktlen] -> spead_pack3/7(hdr_pkt_len_words)
  Assert1/1 -> fifo2/1(data80), fifo3/1(data80)
  spead_pack3/4(data_overflow) -> Terminator2/1
  [adc_data_offset] -> spead_pack2/11(hdr8_0x3300)
  [adc_data_offset] -> spead_pack3/11(hdr8_0x3300)
  spead_pack2/4(data_overflow) -> Terminator1/1
  spead_pack2/3(eof) -> pipeline61/1(d)
  spead_pack2/1(data_out) -> pipeline53/1(d)  "packd"
  spead_pack2/2(valid_out) -> pipeline60/1(d)  "packv"
  spead_pack3/1(data_out) -> pipeline62/1(d)
  spead_pack3/2(valid_out) -> pipeline63/1(d)
  spead_pack3/3(eof) -> pipeline64/1(d)
  pipeline53/1(q) -> [spead_data2]
  pipeline60/1(q) -> [spead_valid2]  "sp_dv0"
  pipeline61/1(q) -> [spead_eof2]
  pipeline62/1(q) -> [spead_data3]
  pipeline63/1(q) -> [spead_valid3]  "sp_dv1"
  pipeline64/1(q) -> [spead_eof3]
  pipeline66/1(q) -> pack_80_64_2/2(valid80)
  pipeline67/1(q) -> pack_80_64_2/3(word_start)
  pipeline68/1(q) -> Delay9/1, pack_80_64_2/4(pkt_start)
  pipeline46/1(q) -> pack_80_64_3/2(valid80)
  pipeline47/1(q) -> pack_80_64_3/3(word_start)
  pipeline48/1(q) -> Delay10/1, pack_80_64_3/4(pkt_start)
  pipeline49/1(q) -> spead_pack2/1(data64_ready), [rdy2]
  pipeline50/1(q) -> spead_pack2/2(data64_valid), [vld2]
  pipeline51/1(q) -> spead_pack3/1(data64_ready), [rdy3]
  pipeline52/1(q) -> spead_pack3/2(data64_valid), [vld3]
  Inverter1/1 -> fifo3/2(fifo_we_en)
  Mux11/1 -> spead_pack3/3(data64)
  [spead_data2] -> pipeline70/1(d)
  [spead_valid2] -> pipeline71/1(d)
  wr_addr2/1 -> 64_to_1/1  "waddr"
  [spead_valid2] -> pipeline69/1(d), edge_detect14/1, edge_detect16/1(in)
  Constant21/1 -> 64_to_1/6
  Constant25/1 -> 64_to_1/5
  rd_addr2/1 -> Relational9/2, 64_to_1/4  "rdaddr"
  edge_detect14/1 -> wr_addr2/1
  pipeline69/1(q) -> wr_addr2/2
  pipeline70/1(q) -> 64_to_1/2
  pipeline71/1(q) -> 64_to_1/3  "dv64_2"
  64_to_1/1 -> Terminator8/1
  edge_detect16/1(out) -> rd_addr2/1
  Constant56/1 -> Relational9/1
  Relational9/1 -> rd_arm2/2  "rd_done"
  rd_arm2/1 -> rd_addr2/2, pipeline72/1(d)  "rd_en"
  pipeline72/1(q) -> edge_detect15/1(in), pipeline73/1(d)  "dv256"
  edge_detect15/1(out) -> [sp256_eof2]  "eof256_2"
  pipeline73/1(q) -> [sp256_dv2]  "dv256_2"
  64_to_1/2 -> Mux16/3, bram_munge2/1(In1)
  [sp256_eof0] -> rd_arm2/3, rd_arm2/1
  [spead_data1] -> pipeline76/1(d)
  [spead_valid1] -> pipeline77/1(d)
  wr_addr1/1 -> 64_to_2/1  "waddr"
  [spead_valid1] -> pipeline75/1(d), edge_detect17/1, edge_detect19/1(in)
  Constant59/1 -> 64_to_2/6
  Constant60/1 -> 64_to_2/5
  rd_addr1/1 -> Relational10/2, 64_to_2/4  "rdaddr"
  edge_detect17/1 -> wr_addr1/1
  pipeline75/1(q) -> wr_addr1/2
  pipeline76/1(q) -> 64_to_2/2
  pipeline77/1(q) -> 64_to_2/3  "dv64_1"
  64_to_2/1 -> Terminator9/1
  edge_detect19/1(out) -> rd_arm1/3, rd_arm1/1, rd_addr1/1
  Constant61/1 -> Relational10/1
  Relational10/1 -> rd_arm1/2  "rd_done"
  rd_arm1/1 -> rd_addr1/2, pipeline78/1(d)  "rd_en"
  pipeline78/1(q) -> edge_detect18/1(in), pipeline79/1(d)  "dv256"
  edge_detect18/1(out) -> [sp256_eof1]  "eof256_1"
  pipeline79/1(q) -> [sp256_dv1]  "dv256_1"
  64_to_2/2 -> Mux18/3, bram_munge1/1(In1)
  [spead_data3] -> pipeline82/1(d)
  [spead_valid3] -> pipeline83/1(d)
  wr_addr3/1 -> 64_to_3/1  "waddr"
  [spead_valid3] -> edge_detect22/1(in), edge_detect20/1, pipeline81/1(d)
  Constant62/1 -> 64_to_3/6
  Constant63/1 -> 64_to_3/5
  rd_addr3/1 -> 64_to_3/4, Relational11/2  "rdaddr"
  edge_detect20/1 -> wr_addr3/1
  pipeline81/1(q) -> wr_addr3/2
  pipeline82/1(q) -> 64_to_3/2
  pipeline83/1(q) -> 64_to_3/3  "dv64_3"
  64_to_3/1 -> Terminator10/1
  edge_detect22/1(out) -> rd_addr3/1
  Constant64/1 -> Relational11/1
  Relational11/1 -> rd_arm3/2  "rd_done"
  rd_arm3/1 -> pipeline84/1(d), rd_addr3/2  "rd_en"
  pipeline84/1(q) -> pipeline85/1(d), edge_detect21/1(in)  "dv256"
  edge_detect21/1(out) -> [sp256_eof3]  "eof256_3"
  pipeline85/1(q) -> [sp256_dv3]  "dv256_3"
  [sp256_eof1] -> rd_arm3/1, rd_arm3/3
  ramp2/1 -> [rampdata2]
  [vld2] -> ramp2/2
  [rdy2] -> ramp2/1
  ramp3/1 -> [rampdata3]
  [vld3] -> ramp3/2
  [rdy3] -> ramp3/1
  [sp256_dv0] -> Mux/1
  [sp256_data0] -> Mux/3
  [sp256_data2] -> Mux/2
  [sp256_dv1] -> pipeline105/1(d)
  Mux/1 -> Mux1/2
  [sp256_data1] -> pipeline87/1(d)
  [sp256_dv3] -> pipeline106/1(d)
  Mux1/1 -> Mux2/2
  [sp256_data3] -> pipeline88/1(d)
  Mux2/1 -> [sp256_data]
  pipeline87/1(q) -> Mux1/3
  pipeline88/1(q) -> pipeline89/1(d)
  pipeline89/1(q) -> Mux2/3
  [sp256_dvg0] -> Logical9/1
  [sp256_dvg1] -> Logical9/2
  [sp256_dvg2] -> Logical9/3
  [sp256_dvg3] -> Logical9/4
  Logical9/1 -> pipeline93/1(d)
  pipeline93/1(q) -> pipeline94/1(d)
  pipeline94/1(q) -> [sp256_dv]
  [sp256_eofg0] -> Logical10/1
  [sp256_eofg1] -> Logical10/2
  [sp256_eofg2] -> Logical10/3
  [sp256_eofg3] -> Logical10/4
  Logical10/1 -> pipeline95/1(d)
  pipeline95/1(q) -> pipeline104/1(d)
  pipeline104/1(q) -> [sp256_eof]  "tx_eof"
  [sp256_dv0] -> Mux5/1
  [gbe_ip0] -> Mux5/3
  [gbe_ip2] -> Mux5/2
  [sp256_dv1] -> Mux6/1
  Mux5/1 -> Mux6/2
  [gbe_ip1] -> pipeline90/1(d)
  [sp256_dv3] -> Mux7/1
  Mux6/1 -> Mux7/2
  [gbe_ip3] -> pipeline91/1(d)
  Mux7/1 -> [gbe_txip]
  pipeline90/1(q) -> Mux6/3
  pipeline91/1(q) -> pipeline92/1(d)
  pipeline92/1(q) -> Mux7/3
  [gbe_txen0] -> Logical11/2
  pipeline43/1(q) -> [sp256_dv0]  "dv256_0"
  [sp256_eof0] -> Logical11/1
  [sp256_dv0] -> Logical12/1
  [gbe_txen0] -> Logical12/2
  Logical12/1 -> [sp256_dvg0]
  Logical11/1 -> [sp256_eofg0]
  [gbe_txen1] -> Logical13/2
  [sp256_eof1] -> Logical13/1
  [sp256_dv1] -> Logical14/1
  [gbe_txen1] -> Logical14/2
  Logical14/1 -> [sp256_dvg1]
  Logical13/1 -> [sp256_eofg1]
  [gbe_txen2] -> Logical15/2
  [sp256_eof2] -> Logical15/1
  [sp256_dv2] -> Logical16/1
  [gbe_txen2] -> Logical16/2
  Logical16/1 -> [sp256_dvg2]
  Logical15/1 -> [sp256_eofg2]
  [gbe_txen3] -> Logical17/2
  [sp256_eof3] -> Logical17/1
  [sp256_dv3] -> Logical18/1
  [gbe_txen3] -> Logical18/2
  Logical18/1 -> [sp256_dvg3]
  Logical17/1 -> [sp256_eofg3]
  [sp256_dvg0] -> Logical22/1
  [sp256_dvg1] -> Logical20/1
  Logical20/1 -> Logical22/2
  [sp256_dvg3] -> Logical20/3
  [sp256_dvg2] -> Logical20/2
  [sp256_dvg1] -> Logical23/1
  [sp256_dvg0] -> Logical21/1
  Logical21/1 -> Logical23/2
  [sp256_dvg3] -> Logical21/3
  [sp256_dvg2] -> Logical21/2
  [sp256_dvg2] -> Logical25/1
  [sp256_dvg0] -> Logical24/1
  Logical24/1 -> Logical25/2
  [sp256_dvg3] -> Logical24/3
  [sp256_dvg1] -> Logical24/2
  [sp256_dvg3] -> Logical27/1
  [sp256_dvg0] -> Logical26/1
  Logical26/1 -> Logical27/2
  [sp256_dvg2] -> Logical26/3
  [sp256_dvg1] -> Logical26/2
  Logical22/1 -> Logical28/1
  Logical23/1 -> Logical28/2
  Logical25/1 -> Logical28/3
  Logical27/1 -> Logical28/4
  Logical28/1 -> Counter/2  "gbe_dv_error"
  [clr_status] -> Counter/1
  Counter/1 -> gbe_valid_err/1(out_reg)
  Constant40/1 -> gbecontrol/2(sim_2)
  Constant23/1 -> gbecontrol/1(sim_1)
  Constant41/1 -> gbecontrol/3(sim_3)
  Constant55/1 -> gbecontrol/4(sim_4)
  pipeline105/1(q) -> Mux1/1
  pipeline106/1(q) -> pipeline107/1(d)
  pipeline107/1(q) -> Mux2/1
  ramp80/1 -> [ramp79]
  [rst_ramp80] -> ramp80/1
  Delay5/1 -> [sel_ramp80]
  test_control/1(in_sel_ramp80) -> Delay5/1
  Delay6/1 -> [rst_ramp80]
  test_control/2(in_rst_ramp80) -> Delay6/1
  [rampdata0] -> Mux8/2
  [sel_ramp80] -> Mux8/1
  pack_80_64_00/3(data64) -> pipeline108/1(d)
  pipeline108/1(q) -> Mux8/3
  [rampdata1] -> Mux9/2
  [sel_ramp80] -> Mux9/1
  pipeline109/1(q) -> Mux9/3
  pack_80_64_1/3(data64) -> pipeline109/1(d)  "d64_00"
  [rampdata2] -> Mux10/2
  [sel_ramp80] -> Mux10/1
  pipeline110/1(q) -> Mux10/3
  [rampdata3] -> Mux11/2
  [sel_ramp80] -> Mux11/1
  pipeline111/1(q) -> Mux11/3
  pack_80_64_3/3(data64) -> pipeline111/1(d)
  pack_80_64_2/3(data64) -> pipeline110/1(d)
  Mux10/1 -> spead_pack2/3(data64)
  Delay7/1 -> Mux12/1
  [speadtime0] -> Mux12/3
  Mux12/1 -> pack_80_64_00/1(data80)  "d80_in"
  Delay8/1 -> Mux13/1
  [speadtime1] -> Mux13/3
  Mux13/1 -> pack_80_64_1/1(data80)
  [ramp79] -> bus_create4/2(in2)  "d80_0"
  Constant1/1 -> bus_create4/1(in1)
  [ramp79] -> bus_create5/2(in2)  "d80_0"
  Constant18/1 -> bus_create5/1(in1)
  Delay9/1 -> Mux14/1
  [speadtime0] -> Mux14/3
  Mux14/1 -> pack_80_64_2/1(data80)
  pipeline65/1(q) -> Mux14/2
  Delay10/1 -> Mux15/1
  [speadtime1] -> Mux15/3
  Mux15/1 -> pack_80_64_3/1(data80)
  pipeline45/1(q) -> Mux15/2
  bus_expand/1(msb_out4) -> ?  "tx_d3"
  bus_expand/2(out3) -> ?  "tx_d2"
  bus_expand/3(out2) -> ?  "tx_d1"
  Constant46/1 -> Relational12/1
  Relational12/1 -> Inverter3/1
  Inverter3/1 -> Logical29/2
  [sp256_eof] -> Logical29/1
  bus_expand/4(lsb_out1) -> Relational12/2  "tx_d0"
  [clr_status] -> Counter1/1
  Counter1/1 -> gbe_last_value_err/1(out_reg)
  Logical29/1 -> Counter1/2  "last_value_error"
  [sp256_data] -> bus_expand/1(bus_in)
  64_to_256/2 -> Mux19/3, bram_munge0/1(In1)
  Delay11/1 -> [sel_munge]
  test_control/3(in_sel_munge) -> Delay11/1
  [sel_munge] -> Mux17/1
  Mux17/1 -> [sp256_data3]
  64_to_3/2 -> Mux17/3, bram_munge3/1(In1)
  [sel_munge] -> Mux16/1
  Mux16/1 -> [sp256_data2]
  [sel_munge] -> Mux18/1
  Mux18/1 -> [sp256_data1]
  [sel_munge] -> Mux19/1
  Mux19/1 -> [sp256_data0]
  bram_munge1/1(Out1) -> Mux18/2
  bram_munge0/1(Out1) -> Mux19/2
  bram_munge2/1(Out1) -> Mux16/2
  bram_munge3/1(Out1) -> Mux17/2
  [gbe_rst] -> forty_gbe/1(rst)
  Constant32/1 -> forty_gbe/7(rx_ack)
  Constant35/1 -> forty_gbe/8(rx_overrun_ack)
  Constant37/1 -> forty_gbe/9(debug_rst)
  [sp256_eof] -> forty_gbe/6(tx_end_of_frame)
  [sp256_dv] -> forty_gbe/3(tx_valid)
  [sp256_data] -> forty_gbe/2(tx_data)
  [gbe_port] -> forty_gbe/5(tx_dest_port)
  [gbe_txip] -> forty_gbe/4(tx_dest_ip)
